simulink model "short_circuit_test_of_3_ph_transformer"  (R2014b)
settings: Solver=ode23tb  StartTime=0.0  StopTime=0.2  MaxStep=1e-4  RelTol=1e-3
libraries: powerlib x7, powerlib_meascontrol x3
settings Model: Creator=Amr Saleh  LastModifiedBy=Amr Saleh

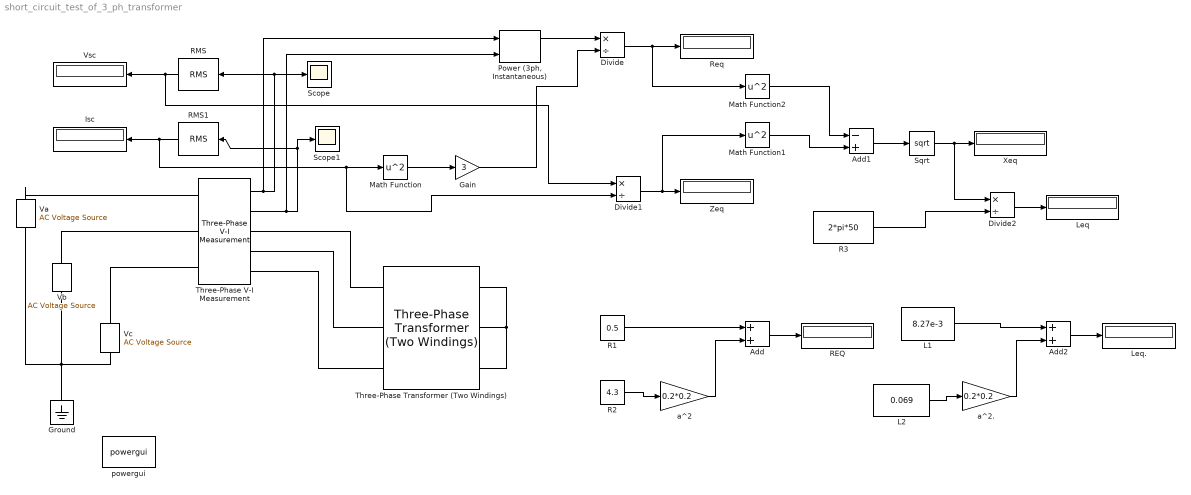
== system short_circuit_test_of_3_ph_transformer ==
  Add : Sum
  Add1 : Sum  Inputs=-+
  Add2 : Sum
  Divide : Product  Inputs=*/
  Divide1 : Product  Inputs=*/
  Divide2 : Product  Inputs=*/
  Gain : Gain  Gain=3
  Ground : powerlib/Elements/Ground  LConnTagsString=a
  Isc : Display
  L1 : Constant  Value=8.27e-3
  L2 : Constant  Value=0.069
  Leq : Display
  Leq. : Display
  Math Function : Math  Operator=square  SaturateOnIntegerOverflow=on
  Math Function1 : Math  Operator=square  SaturateOnIntegerOverflow=on
  Math Function2 : Math  Operator=square  SaturateOnIntegerOverflow=on
  "Power (3ph, Instantaneous)" : powerlib_meascontrol/Measurements/Power (3ph, Instantaneous)
  R1 : Constant  Value=0.5
  R2 : Constant  Value=4.3
  R3 : Constant  Value=2*pi*50
  REQ : Display
  RMS : powerlib_meascontrol/Measurements/RMS  TrueRMS=off  Freq=50  RMSInit=0  Ts=0
  RMS1 : powerlib_meascontrol/Measurements/RMS  TrueRMS=off  Freq=50  RMSInit=0  Ts=0
  Req : Display
  Scope : Scope
  Scope1 : Scope
  Sqrt : Sqrt  SaturateOnIntegerOverflow=on
  Three-Phase Transformer (Two Windings) : powerlib/Elements/Three-Phase Transformer (Two Windings)  Winding1Connection=Y  UNITS=SI  NominalPower=[ 2000e3 , 50 ]  Winding1=[6.6e3 0.5 8.27e-3]  Winding2Connection=Y  Winding2=[33e3 4.3 0.069]  SetSaturation=off  Rm=10000  Lm=500  Saturation=[0 0;0.59382 20.584;247.42 26.073]  Hysteresis=off  DataFile='hysteresis'  SetInitialFlux=off  InitialFluxes=[13.723 -13.723 12.007]  Measurements=None  MoreParameters=off  BreakLoop=off  DataType=on  TransfoNumber=1
  Three-Phase V-I Measurement : powerlib/Measurements/Three-Phase V-I Measurement  VoltageMeasurement=phase-to-ground  SetLabelV=off  LabelV=Vabc  Vpu=off  VpuLL=off  CurrentMeasurement=yes  SetLabelI=off  LabelI=Iabc  Ipu=off  Pbase=100e6  Vbase=500e3  OutputType=Complex  PhasorSimulation=off  PSBequivalent=0
  Va : powerlib/Electrical Sources/AC Voltage Source  Amplitude=0.5*1000*sqrt(2)/sqrt(3)  Phase=0  Frequency=50  SampleTime=0  Measurements=None
  Vb : powerlib/Electrical Sources/AC Voltage Source  Amplitude=0.5*1000*sqrt(2)/sqrt(3)  Phase=-120  Frequency=50  SampleTime=0  Measurements=None
  Vc : powerlib/Electrical Sources/AC Voltage Source  Amplitude=0.5*1000*sqrt(2)/sqrt(3)  Phase=120  Frequency=50  SampleTime=0  Measurements=None
  Vsc : Display
  Xeq : Display
  Zeq : Display
  a^2 : Gain  Gain=0.2*0.2
  a^2. : Gain  Gain=0.2*0.2
  powergui : powerlib/powergui  Priority=1  SimulationMode=Continuous  SolverType=Tustin/Backward Euler (TBE)  SampleTime=50e-6  frequency=60  SPID=off  DisableSnubberDevices=off  DisableRonSwitches=off  DisableVfSwitches=off  SwTol=0  DisplayEquations=off  Interpol=off  methode=off  Ts=100  frequencyindice=50  Pbase=100e6  ErrMax=1e-4  Iterations=50  UnitsV=kV  UnitsW=MW  FunctionMessages=off  echomessages=off  HookPort=off  EnableUseOfTLC=off  x0status=blocks  RestoreLinks=warning  ResistiveCurrentMeasurement=off  Frange=[0:2:500]  Ylog=off  Xlog=on  ShowGrid=off  save=off  variable=ZData  structure=0  ZoomFFT=off  StartTime=0.0  cycles=1  DisplayStyle=1  fundamental=60  FreqAxis=off  MaxFrequency=1000  frequencyindicesteady=1  RmsSteady=1  display=off
  wires:
  Three-Phase V-I Measurement/1 -> "Power (3ph, Instantaneous)"/1, Scope/1, RMS/1
  Three-Phase V-I Measurement/2 -> Scope1/1, RMS1/1, "Power (3ph, Instantaneous)"/2
  RMS/1 -> Divide1/1, Vsc/1
  RMS1/1 -> Divide1/2, Math Function/1, Isc/1
  "Power (3ph, Instantaneous)"/1 -> Divide/1
  Gain/1 -> Divide/2
  Math Function/1 -> Gain/1
  Divide/1 -> Math Function2/1, Req/1
  R1/1 -> Add/1
  R2/1 -> a^2/1
  a^2/1 -> Add/2
  Add/1 -> REQ/1
  Divide1/1 -> Math Function1/1, Zeq/1
  Math Function1/1 -> Add1/2
  Math Function2/1 -> Add1/1
  Add1/1 -> Sqrt/1
  Sqrt/1 -> Divide2/1, Xeq/1
  R3/1 -> Divide2/2
  Divide2/1 -> Leq/1
  L1/1 -> Add2/1
  L2/1 -> a^2./1
  a^2./1 -> Add2/2
  Add2/1 -> Leq./1
  connections:
  Vc/LConn1 -- Ground/LConn1 -- Va/LConn1 -- Vb/LConn1
  Va/RConn1 -- Three-Phase V-I Measurement/LConn1
  Three-Phase V-I Measurement/LConn2 -- Vb/RConn1
  Vc/RConn1 -- Three-Phase V-I Measurement/LConn3
  Three-Phase V-I Measurement/RConn1 -- Three-Phase Transformer (Two Windings)/LConn1
  Three-Phase V-I Measurement/RConn2 -- Three-Phase Transformer (Two Windings)/LConn2
  Three-Phase V-I Measurement/RConn3 -- Three-Phase Transformer (Two Windings)/LConn3
  Three-Phase Transformer (Two Windings)/RConn1 -- Three-Phase Transformer (Two Windings)/RConn2 -- Three-Phase Transformer (Two Windings)/RConn3
